simulink library "DrivingCycle"  (R2023b)
settings: Solver=VariableStepAuto  StartTime=0.0  StopTime=1800  RelTol=1e-3
undefined symbols (not defined in the file or in its folder): h
settings Model: Creator=dadikozyanaa  LastModifiedBy=koenjacobs
settings DebuggingCC: UnconnectedInputMsg=warning  UnconnectedOutputMsg=warning  UnconnectedLineMsg=warning
settings ModelReferenceCC: EnableRefExpFcnMdlSchedulingChecks=on
settings RTWCC: DLArmComputeVersion=19.05

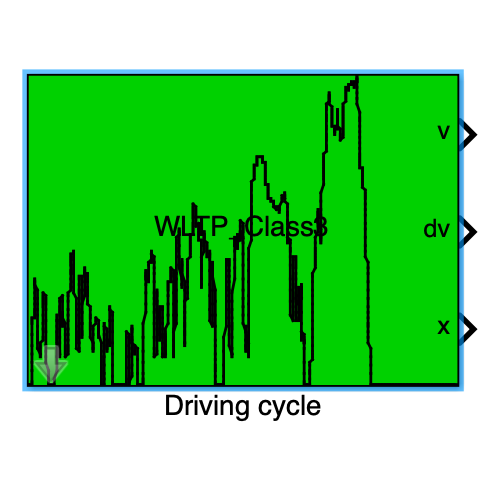
[thumbnail: Simulink's stored preview of the top-level diagram]
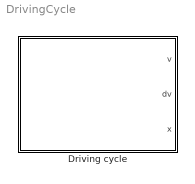
== system DrivingCycle ==
  Driving cycle : Subsystem  mask(Driving cycle){bool_combine=off, cyclenr=Europe: WLTP Class 3, cyclenr2=Europe: EUDC, gradient_speed=0, cyclerep=1, stepsize=1, autostop=on, slope_bool_cycle=on, mode_bool=off, mode_array=0}
      mask prompts: bool_combine "Combine two driving cycles"; cyclenr "Choose a driving cycle:"; cyclenr2 "Choose a second driving cycle:"; gradient_speed "Enter velocity for gradiet test [km/h]:"; cyclerep "Choose cycle repetitions:"; stepsize "Step size:"; autostop "Enable automatic simulation stop"; slope_bool_cycle "Include road slope from cycle"; mode_bool "Include mode associated with cycle"; mode_array "Enter mode array:"
      mask help:
      | Output:
      | =====
      | 	v	Speed [m/s]
      | 	dv	Acceleration [m/s^2]
      | 	slope	Road slope [rad] (optional)
      | 	x	Total distance [m]
      | 	mode	Mode associated with cycle [-] (optional)
      |
      | Enable automatic simulation stop:
      | =====
      | Stops the simulation automatically at the end of the cycle.
      | Be careful: If you have a component in your model that has to run after the cycle has finished, e.g. a battery to charge, remove the mark!
      mask init:
      | init_driving_cycle;
      | %%
      | slope = find_system(gcb, 'LookUnderMasks','on', 'FollowLinks','on', 'Name','slope');
      | mode = find_system(gcb, 'LookUnderMasks','on', 'FollowLinks','on', 'Name','mode');
      | %%
      | % if(slope_bool_cycle)
      | %     if isempty(slope)
      | %         if ~isempty(mode)
      | %         	set_param([gcb,'/mode'],'port','5');
      | %         end
      | %         set_param([gcb,'/x'],'port','4');
      | %         add_block('built-in/Outport',[gcb,'/slope']);
      | %         set_param([gcb,'/slope'],'Position',[490   188   520   212]);     
      | %         add_line(gcb,['slope_cycle/1'],['slope/1']);
      | %         add_block('simulink/Sinks/To Workspace',[gcb,'/Output_slope'],'Saveformat','Array','SampleTime','-1','VariableName','slope','MaxDataPoints','inf');
      | %         set_param([gcb,'/Output_slope'],'Position',[555   220   605   240]);  
      | %         add_line(gcb,'slope_cycle/1','Output_slope/1');
      | %     end
      | % else
      | %     if ~isempty(slope)
      | %         delete_line(gcb,'slope_cycle/1','slope/1');
      | %         delete_line(gcb,'slope_cycle/1','Output_slope/1');
      | %         delete_block([gcb,'/Output_slope']);
      | %         delete_block(slope);
      | %         %delete_line(find_system(gcb, 'FindAll', 'on', 'Type', 'line', 'Connected', 'off'));
      | %     end
      | % end
      | %%
      | if(mode_bool)
      |     if isempty(mode)
      |         add_block('built-in/Outport',[gcb,'/mode']);
      |         add_line(gcb,['Constant_mode/1'],['mode/1']);
      |         add_block('simulink/Sinks/To Workspace',[gcb,'/Output_mode'],'Saveformat','Array','SampleTime','-1','VariableName','mode','MaxDataPoints','inf');
      |         add_line(gcb,'Constant_mode/1','Output_mode/1');
      |     end
      | else
      |     if ~isempty(mode)
      |         delete_line(gcb,'Constant_mode/1','mode/1');
      |         delete_line(gcb,'Constant_mode/1','Output_mode/1');
      |         delete_block([gcb,'/Output_mode']);
      |         delete_block(mode);
      |     end
      | end
      mask Callback bool_combine:
      | maskStr = get_param(gcb,'bool_combine');
      | 
      | p = Simulink.Mask.get(gcb);
      | cycle1 = p.Parameters(2);
      | cycle2 = p.Parameters(3);
      | gradient = p.Parameters(4);
      | repetitions = p.Parameters(5);
      | slope_set = p.Parameters(8);
      | 
      | if strcmp(maskStr, 'on')
      |     cycle1.TypeOptions = {"Europe: WLTP Class 1", "Europe: WLTP Class 2", "Europe: WLTP Class 3",...
      |     "Europe: ECE", "Europe: ECE R15 spez", "Europe: EUDC", "Europe: City", "Europe: NEDC",...
      |     "Europe: VECTO Delivery", "Europe: VECTO Long haul", "Europe: VECTO Municipal", "Japan:  10-15-Mode",...
      |     "Japan:  10-Mode", "Japan:  10-Mode-3", "Japan:  11-Mode", "Japan:  11-Mode-4", "Japan:  15-Mode",...
      |     "USA:    City-I", "USA:    City-II", "USA:    FTP-75", "USA:    FTP-Highway"};
      |     cycle2.Visible = 'on';
      |     gradient.set('Visible','off');
      |     repetitions.set('Enabled','on');
      |     repetitions.Value = '1';
      |     slope_set.Enabled = 'on';
      | else
      |     cycle1.TypeOptions = {"Europe: WLTP Class 1", "Europe: WLTP Class 2", "Europe: WLTP Class 3",...
      |     "Europe: ECE", "Europe: ECE R15 spez", "Europe: EUDC", "Europe: City", "Europe: NEDC",...
      |     "Europe: VECTO Delivery", "Europe: VECTO Long haul", "Europe: VECTO Municipal", "Japan:  10-15-Mode",...
      |     "Japan:  10-Mode", "Japan:  10-Mode-3", "Japan:  11-Mode", "Japan:  11-Mode-4", "Japan:  15-Mode",...
      |     "USA:    City-I", "USA:    City-II", "USA:    FTP-75", "USA:    FTP-Highway"};
      |     cycle2.Visible = 'off';
      | end
      mask TypeOptions cyclenr: Europe: WLTP Class 1 | Europe: WLTP Class 2 | Europe: WLTP Class 3 | Europe: ECE | Europe: ECE R15 spez | Europe: EUDC | Europe: City | Europe: NEDC | Europe: VECTO Delivery | Europe: VECTO Long haul | Europe: VECTO Municipal | Japan:  10-15-Mode | Japan:  10-Mode | Japan:  10-Mode-3 | Japan:  11-Mode | Japan:  11-Mode-4 | Japan:  15-Mode | USA:    City-I | USA:    City-II | USA:    FTP-75 | USA:    FTP-Highway
      mask Callback cyclenr:
      | maskStr = get_param(gcb,'cyclenr');
      | 
      | p = Simulink.Mask.get(gcb);
      | gradient = p.Parameters(4);
      | repetitions = p.Parameters(5);
      | slope_set = p.Parameters(8);
      | timestep = p.Parameters(6);
      | 
      | if strcmp(maskStr, 'Test:    Gradient (specify speed)')
      |     repetitions.Enabled = 'off';
      |     repetitions.Value = '1';
      |     gradient.Visible = 'on';
      |     slope_set.Value = 'on';
      |     slope_set.Enabled = 'off';
      |     timestep.Enabled = 'off';
      |     timestep.Value = '1';
      | elseif strcmp(maskStr, 'Test:    Gradient (standstill)')
      |     repetitions.Enabled = 'off';
      |     repetitions.Value = '1';
      |     gradient.Visible = 'off';
      |     slope_set.Value = 'on';
      |     slope_set.Enabled = 'off';
      |     timestep.Enabled = 'off';
      |     timestep.Value = '1';
      | elseif strcmp(maskStr, 'Test:    Top speed')
      |     repetitions.Enabled = 'off';
      |     repetitions.Value = '1';
      |     gradient.Visible = 'off';
      |     slope_set.Enabled = 'on';
      |     timestep.Enabled = 'off';
      |     timestep.Value = '1';
      | else
      |     gradient.Visible = 'off';
      |     repetitions.Enabled = 'on';
      |     slope_set.Enabled = 'on';
      |     timestep.Enabled = 'on';
      | end
      mask TypeOptions cyclenr2: Europe: WLTP Class 1 | Europe: WLTP Class 2 | Europe: WLTP Class 3 | Europe: ECE | Europe: ECE R15 spez | Europe: EUDC | Europe: City | Europe: NEDC | Europe: VECTO Delivery | Europe: VECTO Long haul | Europe: VECTO Municipal | Japan:  10-15-Mode | Japan:  10-Mode | Japan:  10-Mode-3 | Japan:  11-Mode | Japan:  11-Mode-4 | Japan:  15-Mode | USA:    City-I | USA:    City-II | USA:    FTP-75 | USA:    FTP-Highway
      mask Callback mode_bool:
      | mode_bool = get_param(gcb,'mode_bool');
      | 
      | p = Simulink.Mask.get(gcb);
      | mode = p.Parameters(10);
      | 
      | if strcmp(mode_bool,'on')
      |     mode.set('Visible','on');
      | else
      |     mode.set('Value','0','Visible','off');
      | end
      mask DialogControl Container3 Prompt: Optional settings
      mask Display:
      | plot(T_zplot, V_zplot);
      | disp(cycle_name);

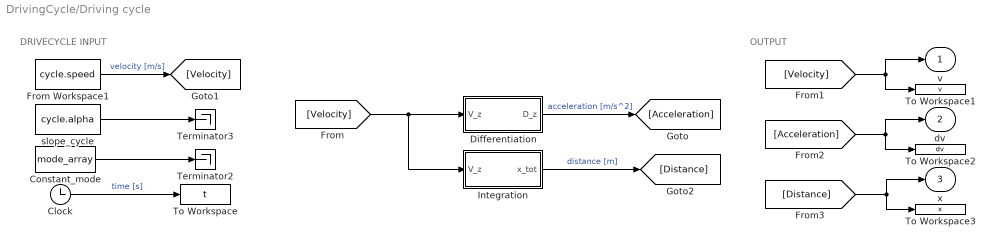
== system DrivingCycle/Driving cycle ==
  note: DRIVECYCLE INPUT
  note: OUTPUT
  Clock : Clock
  Constant_mode : Constant  Value=mode_array
  Differentiation : Subsystem
  From Workspace1 : FromWorkspace  VariableName=cycle.speed
  Integration : Subsystem
  Terminator2 : Terminator
  Terminator3 : Terminator
  To Workspace : ToWorkspace  VariableName=t  SampleTime=-1
  To Workspace1 : ToWorkspace  VariableName=v  SampleTime=-1
  To Workspace2 : ToWorkspace  VariableName=dv  SampleTime=-1
  To Workspace3 : ToWorkspace  VariableName=x  SampleTime=-1
  slope_cycle : FromWorkspace  VariableName=cycle.alpha
  v : Outport
  dv : Outport  Port=2
  x : Outport  Port=3
  wires:
  Constant_mode/1 -> Terminator2/1
  Clock/1 -> To Workspace/1  "time [s]"
  slope_cycle/1 -> Terminator3/1
  From Workspace1/1 -> [Velocity]  "velocity [m/s]"
  Integration/1(x_tot) -> [Distance]  "distance [m]"
  Differentiation/1(D_z) -> [Acceleration]  "acceleration [m/s^2]"
  [Velocity] -> Integration/1(V_z), Differentiation/1(V_z)
  [Distance] -> To Workspace3/1, x/1
  [Acceleration] -> To Workspace2/1, dv/1
  [Velocity] -> v/1, To Workspace1/1

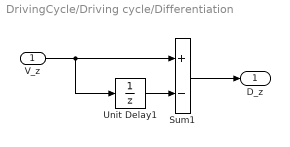
== system DrivingCycle/Driving cycle/Differentiation ==
  V_z : Inport
  Sum1 : Sum  Inputs=+-  InputSameDT=on  SaturateOnIntegerOverflow=on  OutDataTypeStr=Inherit: Same as first input
  Unit Delay1 : UnitDelay  SampleTime=h
  D_z : Outport  InitialOutput=0
  wires:
  Unit Delay1/1 -> Sum1/2
  V_z/1 -> Sum1/1, Unit Delay1/1
  Sum1/1 -> D_z/1

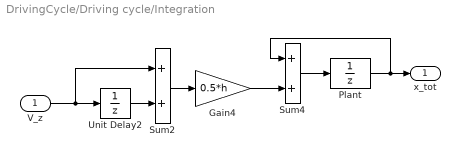
== system DrivingCycle/Driving cycle/Integration ==
  V_z : Inport
  Gain4 : Gain  Gain=0.5*h  SaturateOnIntegerOverflow=on  OutDataTypeStr=Inherit: Same as input  ParamDataTypeStr=Inherit: Same as input
  Plant : UnitDelay  InitialCondition=1  SampleTime=h
  Sum2 : Sum  InputSameDT=on  SaturateOnIntegerOverflow=on  OutDataTypeStr=Inherit: Same as first input
  Sum4 : Sum  InputSameDT=on  SaturateOnIntegerOverflow=on  OutDataTypeStr=Inherit: Same as first input
  Unit Delay2 : UnitDelay  SampleTime=h
  x_tot : Outport  InitialOutput=0
  wires:
  Sum2/1 -> Gain4/1
  Unit Delay2/1 -> Sum2/2
  V_z/1 -> Sum2/1, Unit Delay2/1
  Gain4/1 -> Sum4/2
  Sum4/1 -> Plant/1
  Plant/1 -> Sum4/1, x_tot/1
